simulink model "Forces_Verfication"  (R2018b)
settings: Solver=VariableStepAuto  StartTime=0.0  StopTime=10.0  RelTol=1e-3
InitFcn:
  | Sim_Parameters;
  | Missile_Data;
values from neighbouring files (symbols this model uses):
  D = 0.150    (= 0.15)    [Missile_Data.m]
  Mass = 30.0    (= 30)    [Missile_Data.m]
  S = ( pi / 4 ) * D^2    (= 0.0176714586764)    [Missile_Data.m]
undefined symbols (not defined in the file or in its folder): UNIT_GRAV
libraries: aerolibatmos2 x1, sharedtransform x1
settings Model: Creator=auten  LastModifiedBy=auten

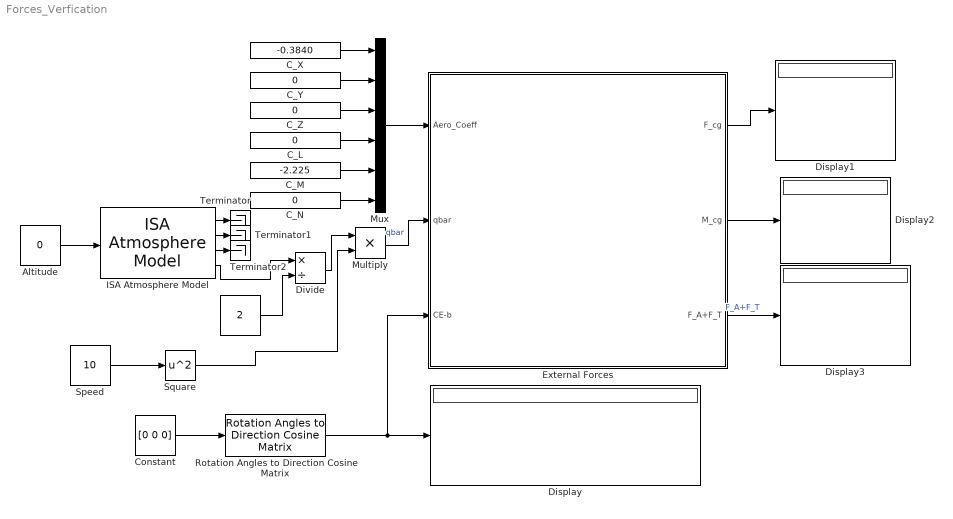
== system Forces_Verfication ==
  " " : Constant  Value=2  VectorParams1D=off  SampleTime=-1
  Altitude : Constant  Value=0  VectorParams1D=off  SampleTime=-1
  C_L : Constant  Value=0  VectorParams1D=off  SampleTime=-1
  C_M : Constant  Value=-2.225  VectorParams1D=off  SampleTime=-1
  C_N : Constant  Value=0  VectorParams1D=off  SampleTime=-1
  C_X : Constant  Value=-0.3840  VectorParams1D=off  SampleTime=-1
  C_Y : Constant  Value=0  VectorParams1D=off  SampleTime=-1
  C_Z : Constant  Value=0  VectorParams1D=off  SampleTime=-1
  Constant : Constant  Value=[0 0 0]  VectorParams1D=off  SampleTime=-1
  Display{,1..3} (4 alike) : Display
  Divide : Product  Inputs=*/
  External Forces : Subsystem
  ISA Atmosphere Model : aerolibatmos2/ISA Atmosphere Model  custom=off  g=9.80665  gamma=1.4  R=287.0531  L=0.0065  h_trop=11000  h_strat=20000  rho0=1.225  P0=101325  T0=288.15  h0=0
      settings: SourceProductName=Aerospace Blockset
  Multiply : Product
  Mux : Mux  Inputs=6
  Rotation Angles to Direction Cosine Matrix : sharedtransform/Rotation Angles to Direction Cosine Matrix  rotationOrder=ZYX  aMode=aMode
      settings: SourceProductBaseCode=AE
  Speed : Constant  Value=10  VectorParams1D=off  SampleTime=-1
  Square : Math  Operator=square  SaturateOnIntegerOverflow=on
  Terminator : Terminator
  Terminator1 : Terminator
  Terminator2 : Terminator
  wires:
  Mux/1 -> External Forces/1(Aero_Coeff)
  C_X/1 -> Mux/1
  C_N/1 -> Mux/6
  C_M/1 -> Mux/5
  C_L/1 -> Mux/4
  C_Y/1 -> Mux/2
  C_Z/1 -> Mux/3
  ISA Atmosphere Model/4 -> Divide/1
  ISA Atmosphere Model/1 -> Terminator/1
  ISA Atmosphere Model/2 -> Terminator1/1
  ISA Atmosphere Model/3 -> Terminator2/1
  Altitude/1 -> ISA Atmosphere Model/1
  " "/1 -> Divide/2
  Divide/1 -> Multiply/1
  Speed/1 -> Square/1
  Square/1 -> Multiply/2
  Multiply/1 -> External Forces/2(qbar)  "qbar"
  Constant/1 -> Rotation Angles to Direction Cosine Matrix/1
  Rotation Angles to Direction Cosine Matrix/1 -> External Forces/3(CE-b), Display/1
  External Forces/1(F_cg) -> Display1/1
  External Forces/2(M_cg) -> Display2/1
  External Forces/3(F_A+F_T) -> Display3/1  "F_A+F_T"

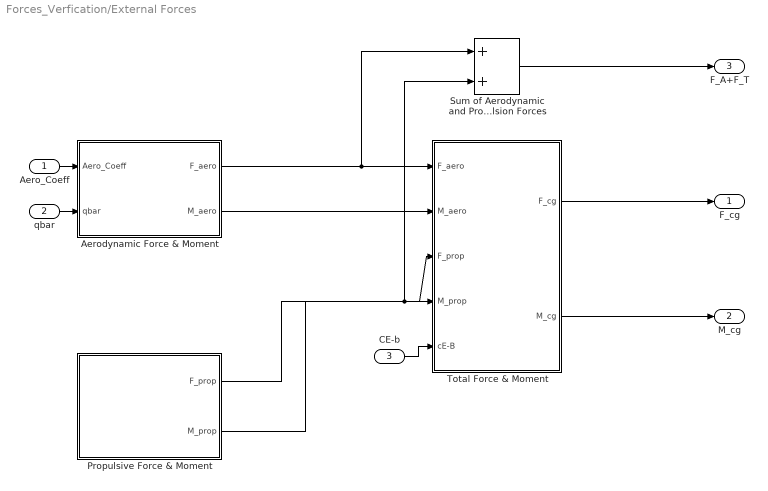
== system Forces_Verfication/External Forces ==
  Aero_Coeff : Inport
  qbar : Inport  Port=2
  CE-b : Inport  Port=3
  Aerodynamic Force & Moment : Subsystem  AncestorBlock=UAS_Model_library/External Forces/Aerodynamics/Aerodynamic Force & Moment
  Propulsive Force & Moment : Subsystem  AncestorBlock=UAS_Model_library/External Forces/Propulsive/Propulsive Force & Moment
  Sum of Aerodynamic and Propulsion Forces : Sum
  Total Force & Moment : Subsystem  AncestorBlock=UAS_Model_library/External Forces/Total Force & Moment
  F_cg : Outport
  M_cg : Outport  Port=2
  F_A+F_T : Outport  Port=3
  wires:
  Total Force & Moment/2(M_cg) -> M_cg/1
  Aerodynamic Force & Moment/2(M_aero) -> Total Force & Moment/2(M_aero)
  Propulsive Force & Moment/2(M_prop) -> Total Force & Moment/4(M_prop)
  Total Force & Moment/1(F_cg) -> F_cg/1
  Aerodynamic Force & Moment/1(F_aero) -> Sum of Aerodynamic and Propulsion Forces/1, Total Force & Moment/1(F_aero)
  Propulsive Force & Moment/1(F_prop) -> Sum of Aerodynamic and Propulsion Forces/2, Total Force & Moment/3(F_prop)
  qbar/1 -> Aerodynamic Force & Moment/2(qbar)
  Aero_Coeff/1 -> Aerodynamic Force & Moment/1(Aero_Coeff)
  Sum of Aerodynamic and Propulsion Forces/1 -> F_A+F_T/1
  CE-b/1 -> Total Force & Moment/5("cE-B ")

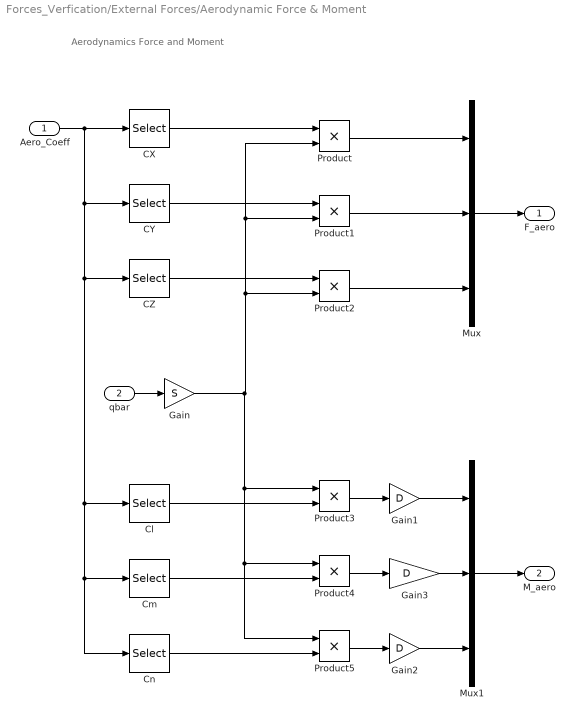
== system Forces_Verfication/External Forces/Aerodynamic Force & Moment ==
  note: Aerodynamics Force and Moment
  Aero_Coeff : Inport
  qbar : Inport  Port=2
  CX : Selector  InputPortWidth=6  IndexOptions=Index vector (dialog)  Indices=[1]  OutputSizes=1
  CY : Selector  InputPortWidth=6  IndexOptions=Index vector (dialog)  Indices=[2]  OutputSizes=1
  CZ : Selector  InputPortWidth=6  IndexOptions=Index vector (dialog)  Indices=[3]  OutputSizes=1
  Cl : Selector  InputPortWidth=6  IndexOptions=Index vector (dialog)  Indices=[4]  OutputSizes=1
  Cm : Selector  InputPortWidth=6  IndexOptions=Index vector (dialog)  Indices=[5]  OutputSizes=1
  Cn : Selector  InputPortWidth=6  IndexOptions=Index vector (dialog)  Indices=[6]  OutputSizes=1
  Gain : Gain  Gain=S
  Gain1 : Gain  Gain=D
  Gain2 : Gain  Gain=D
  Gain3 : Gain  Gain=D
  Mux : Mux  Inputs=3
  Mux1 : Mux  Inputs=3
  Product{,1..5} (6 alike) : Product
  F_aero : Outport
  M_aero : Outport  Port=2
  wires:
  Gain3/1 -> Mux1/2
  Gain2/1 -> Mux1/3
  Gain1/1 -> Mux1/1
  Mux1/1 -> M_aero/1
  Product5/1 -> Gain2/1
  Product4/1 -> Gain3/1
  Product3/1 -> Gain1/1
  Cn/1 -> Product5/2
  Cm/1 -> Product4/2
  Cl/1 -> Product3/2
  Mux/1 -> F_aero/1
  Product2/1 -> Mux/3
  Product1/1 -> Mux/2
  Product/1 -> Mux/1
  CZ/1 -> Product2/1
  CY/1 -> Product1/1
  Gain/1 -> Product/2, Product1/2, Product2/2, Product3/1, Product4/1, Product5/1
  CX/1 -> Product/1
  qbar/1 -> Gain/1
  Aero_Coeff/1 -> CX/1, CY/1, CZ/1, Cm/1, Cn/1, Cl/1

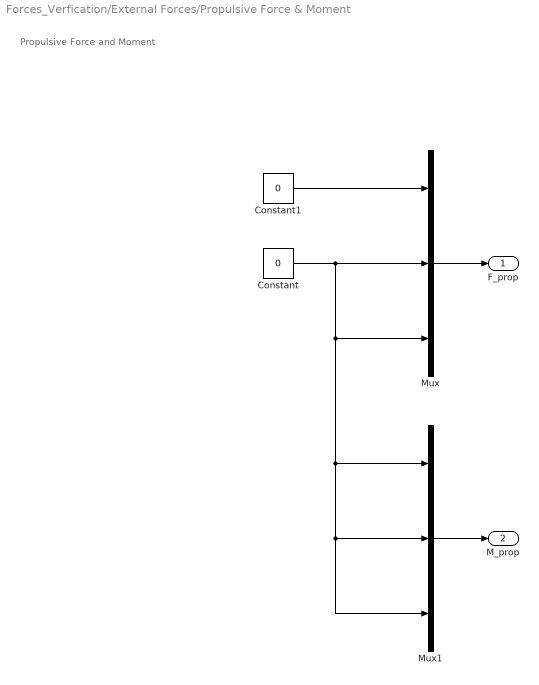
== system Forces_Verfication/External Forces/Propulsive Force & Moment ==
  note: Propulsive Force and Moment
  Constant : Constant  Value=0
  Constant1 : Constant  Value=0
  Mux : Mux  Inputs=3
  Mux1 : Mux  Inputs=3
  F_prop : Outport
  M_prop : Outport  Port=2
  wires:
  Mux/1 -> F_prop/1
  Constant/1 -> Mux/2, Mux1/1, Mux1/2, Mux1/3, Mux/3
  Mux1/1 -> M_prop/1
  Constant1/1 -> Mux/1

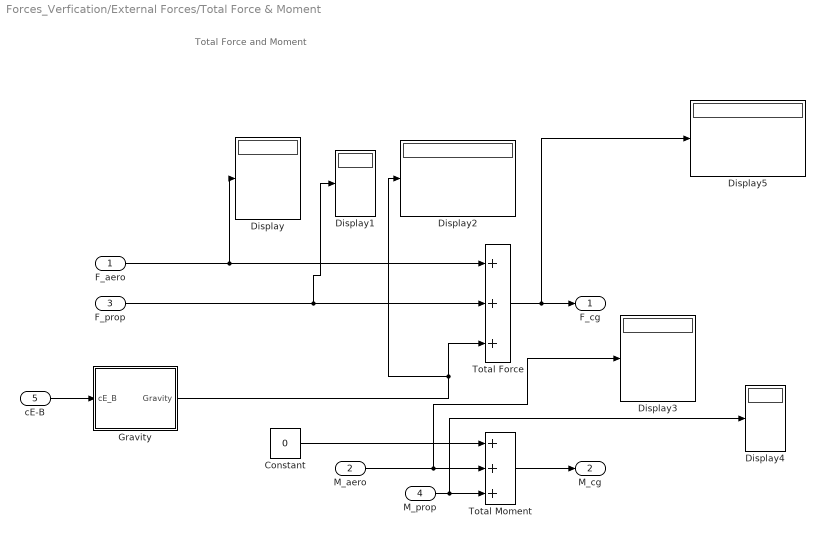
== system Forces_Verfication/External Forces/Total Force & Moment ==
  note: Total Force and Moment
  F_aero : Inport  PortDimensions=3
  M_aero : Inport  Port=2  PortDimensions=3
  F_prop : Inport  Port=3  PortDimensions=3
  M_prop : Inport  Port=4  PortDimensions=3
  "cE-B " : Inport  Port=5
  Constant : Constant  Value=0
  Display{,1..5} (6 alike) : Display
  Gravity : Subsystem  AncestorBlock=UAS_Model_library/Envrionment/Gravity
  Total Force : Sum  Inputs=+++  SaturateOnIntegerOverflow=on  InputSameDT=on  OutDataTypeStr=Inherit: Same as first input
  Total Moment : Sum  Inputs=+++  SaturateOnIntegerOverflow=on  InputSameDT=on  OutDataTypeStr=Inherit: Same as first input
  F_cg : Outport
  M_cg : Outport  Port=2
  wires:
  Gravity/1(Gravity) -> Total Force/3, Display2/1
  Total Moment/1 -> M_cg/1
  M_prop/1 -> Display4/1, Total Moment/3
  F_prop/1 -> Display1/1, Total Force/2
  F_aero/1 -> Display/1, Total Force/1
  Constant/1 -> Total Moment/1
  M_aero/1 -> Display3/1, Total Moment/2
  "cE-B "/1 -> Gravity/1(cE_B)
  Total Force/1 -> Display5/1, F_cg/1

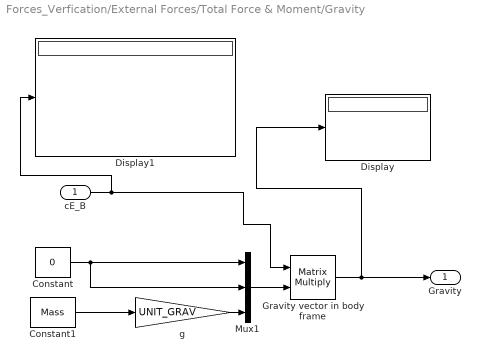
== system Forces_Verfication/External Forces/Total Force & Moment/Gravity ==
  cE_B : Inport
  Constant : Constant  Value=0
  Constant1 : Constant  Value=Mass
  Display : Display
  Display1 : Display
  "Gravity vector in body frame " : Product  Multiplication=Matrix(*)  SaturateOnIntegerOverflow=on  InputSameDT=on  OutDataTypeStr=Inherit: Same as first input
  Mux1 : Mux  Inputs=3
  g : Gain  Gain=UNIT_GRAV
  Gravity : Outport
  wires:
  Constant1/1 -> g/1
  "Gravity vector in body frame "/1 -> Display/1, Gravity/1
  g/1 -> Mux1/3
  Mux1/1 -> "Gravity vector in body frame "/2
  cE_B/1 -> Display1/1, "Gravity vector in body frame "/1
  Constant/1 -> Mux1/1, Mux1/2
